simulink model "V_Curves"  (R2020a)
settings: Solver=VariableStepAuto  StartTime=0.0  StopTime=2  RelTol=1e-3
libraries: powerlib x8, powerlib_meascontrol x3
settings Model: Creator=krishna  LastModifiedBy=krishna

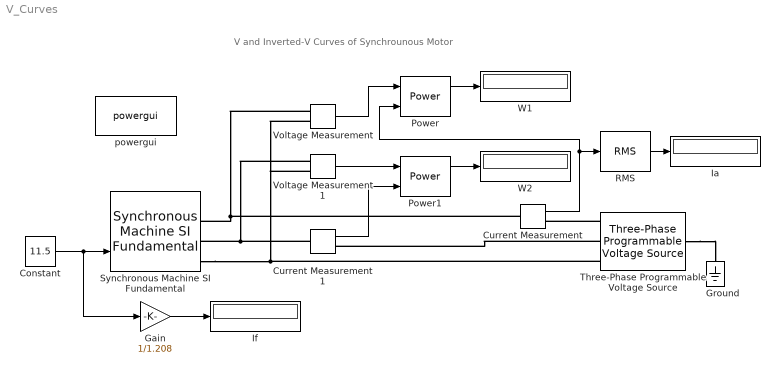
== system V_Curves ==
  note: V and Inverted-V Curves of Synchrounous Motor
  Constant : Constant  Value=11.5
  Current Measurement : powerlib/Measurements/Current Measurement  PhasorSimulation=off  OutputType=Complex  PSBequivalent=0
  Current Measurement1 : powerlib/Measurements/Current Measurement  PhasorSimulation=off  OutputType=Complex  PSBequivalent=0
  Gain : Gain  Gain=1/1.208
  Ground : powerlib/Elements/Ground  LConnTagsString=a
  Ia : Display
  If : Display
  Power : powerlib_meascontrol/Measurements/Power  Freq=50  Vinit=[1, 0]  Iinit=[1, 0]  Ts=0
  Power1 : powerlib_meascontrol/Measurements/Power  Freq=50  Vinit=[1, 0]  Iinit=[1, 0]  Ts=0
  RMS : powerlib_meascontrol/Measurements/RMS  TrueRMS=on  Freq=50  RMSInit=0  Ts=0
  Synchronous Machine SI Fundamental : powerlib/Machines/Synchronous Machine SI Fundamental  PresetModel=01: 50Hz 400V 8.1kVA 1500RPM  MechanicalLoad=Mechanical power Pm  ShowDetailedParameters=on  RotorType=Salient-pole  Units=SI fundamental parameters  MeasurementBus=off  NominalParameters=[8100 400 50]  Stator=[1.62 0.004527 0.1086 0.05175]  Field=[1.208 0.01132]  Dampers2=[ 0.0664, 1.387e-3, 0.0292, 6.896e-4, 7.907e-3, 2.477e-3]  Dampers1=[3.142 0.007334 4.772 0.01015]  Mechanical=[0.0923 0.009 2]  PolePairs=2  InitialConditions="[ 0  0  0  0  0  0  0  0  70.3192 ]"  SetSaturation=off  Saturation=[695.64,774.7,917.5,1001.6,1082.2,1175.9,1293.6,1430.2,1583.7;9660,10623,12243,13063,13757,14437,15180,15890,16567]  DisplayVfd=off  LoadFlowParameters=[1,0,0,0,0]  TsPowergui=0  TsBlock=-1  IterativeModel=Trapezoidal non iterative  IterativeDiscreteModel=Trapezoidal non iterative  BusType=PV  Pref=0  Qref=0  Qmin=-inf  Qmax=inf  PLF=0  QLF=0
      settings: SourceProductBaseCode=PS
  Three-Phase Programmable Voltage Source : powerlib/Electrical Sources/Three-Phase Programmable Voltage Source  PositiveSequence="[400  0 50]"  VariationEntity=None  VariationType=Table of time-amplitude pairs  VariationTypeAlt=Step  VariationStep=0.5  VariationRate=10  VariationMagnitude=0.3  VariationFrequency=2  VariationTiming=[1 2]  VariationPhaseA=off  Amplitudes=[1 0.8 1.2 1.0]  TimeValues=[0 0.1 0.15 0.2]  HarmonicGeneration=off  HarmonicA=[3 0.2 -25 0]  HarmonicB=[2 0.15 35 2]  Timing="[0.05  3]"  BusType=swing  Pref=0  Qref=0  Qmin=-inf  Qmax=inf
  Voltage Measurement : powerlib/Measurements/Voltage Measurement  PhasorSimulation=off  OutputType=Complex  PSBequivalent=0
  Voltage Measurement1 : powerlib/Measurements/Voltage Measurement  PhasorSimulation=off  OutputType=Complex  PSBequivalent=0
  W1 : Display
  W2 : Display
  powergui : powerlib/powergui  Priority=1  SimulationMode=Continuous  SampleTime=50e-6  frequency=60  Iterations=50  frequencyindice=50  Pbase=100e6  ErrMax=1e-4  UnitsV=kV  UnitsW=MW  buscounter=0  FunctionMessages=off  echomessages=off  EnableUseOfTLC=off  CurrentSourceSwitches=off  DisableSnubberDevices=off  DisableRonSwitches=off  DisableVfSwitches=off  DisplayEquations=off  AutomaticDiscreteSolvers=off  SolverType=Tustin/Backward Euler (TBE)  Interpol=off  ExternalGateDelay=off  methode=off  Ts=100  x0status=blocks  SPID=on  SwTol=0  HookPort=off  NonlinearTolerance=1e-4  nMaxIteration=100  ContinueOnMaxIteration=off  RestoreLinks=warning  ResistiveCurrentMeasurement=off  Frange=[0:2:500]  Ylog=off  Xlog=on  ShowGrid=off  save=off  variable=ZData  structure=0  ZoomFFT=off  StartTime=0.0  cycles=1  DisplayStyle=1  fundamental=60  FreqAxis=off  MaxFrequency=1000  frequencyindicesteady=1  RmsSteady=1  display=off
  wires:
  Current Measurement/1 -> Power/2, RMS/1
  RMS/1 -> Ia/1
  Constant/1 -> Gain/1, Synchronous Machine SI Fundamental/2
  Gain/1 -> If/1
  Voltage Measurement/1 -> Power/1
  Voltage Measurement1/1 -> Power1/1
  Current Measurement1/1 -> Power1/2
  Power/1 -> W1/1
  Power1/1 -> W2/1
  connections:
  Voltage Measurement1/LConn1 -- Current Measurement1/LConn1 -- Synchronous Machine SI Fundamental/RConn2
  Synchronous Machine SI Fundamental/RConn3 -- Three-Phase Programmable Voltage Source/RConn3 -- Voltage Measurement/LConn2 -- Voltage Measurement1/LConn2
  Three-Phase Programmable Voltage Source/RConn1 -- Current Measurement/RConn1
  Current Measurement/LConn1 -- Synchronous Machine SI Fundamental/RConn1 -- Voltage Measurement/LConn1
  Three-Phase Programmable Voltage Source/RConn2 -- Current Measurement1/RConn1
  Three-Phase Programmable Voltage Source/LConn1 -- Ground/LConn1
